simulink library "SDTlibV1"  (R2025b)
settings: Solver=VariableStepAuto  StartTime=0.0  StopTime=10.0  RelTol=1e-3
PreLoadFcn:
  | addpath(genpath('SDTfct'));
values from neighbouring files (symbols this model uses):
  pass = ra2DCMi(blk.ra)    [view_SDTlib_model.m]
undefined symbols (not defined in the file or in its folder): CMG, DAP0, DPa0, FSM, Ignew, InvDyn, InvDynAug, Jr, KIN, kinematic_model, LS, Mdyn, mnew, mp, OGnew, PMA, ra_norm, RWS, sig4, uls, ureal, uss, uw, XI
libraries: RCTblocks x470, $bdroot x4
(part 1 of 10)
settings Model: Creator=d.alazard  LastModifiedBy=ervan
settings SolverCC: AlgebraicLoopSolver=TrustRegion
settings DataIOCC: ReturnWorkspaceOutputs=off
settings DebuggingCC: UnconnectedInputMsg=warning  UnconnectedOutputMsg=warning  UnconnectedLineMsg=warning  ArithmeticOperatorsInVariantConditions=warning
settings ModelReferenceCC: EnableRefExpFcnMdlSchedulingChecks=on
settings SFSimCC: CustomCodeUndefinedFunction=UseInterfaceOnly
settings RTWCC: GPUComputeCapability=3.5  DLArmComputeVersion=19.05

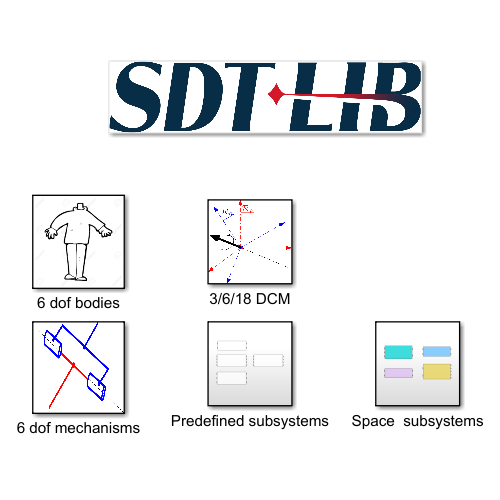
[thumbnail: Simulink's stored preview of the top-level diagram]
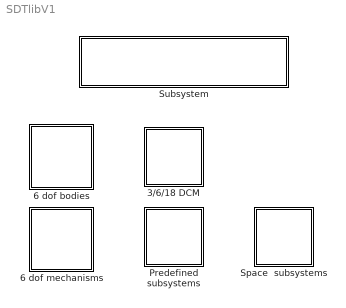
== system SDTlibV1 ==
  3/6/18 DCM : Subsystem
      mask Display: image('logoDCM.png')
  6 dof bodies : Subsystem
      mask Display: image('index.png')
  6 dof mechanisms : Subsystem
      mask Display: image('logomechanisms.png')
  Predefined subsystems : Subsystem
  Space  subsystems : Subsystem
  Subsystem : Subsystem
      mask Display: image('SDTlib_logo.png')

== system SDTlibV1/3//6//18 DCM ==
  18x18 DCM : Subsystem  mask(18x18 Direction cosine matrix (DCM)){rot=[0 1 0;-1 0 0;0 0 1], transp=off}
      mask prompts: rot "3x3 DCM"; transp "Matrix transposed"
      mask help:
      | For 6 d.o.f. body motion vector (3 translations and 3 rotations, accelerations, velocities and positions), this block Implement the 18x18 rotation matrix (or its transposed) for a given 3x3 DCM.
      |
      | Considering 2 frames R1 and  R2, the DCM between R1 and R2 is defined as the 3x3 matrix where each column is the component vector of each R2 orthogonal unit vector expressed in R1. Thus
      |
      |    [v]_R1 = DCM  * [v]_R2.
      mask init:
      | if transp,
      |     rot=rot';
      | end
      mask Help: web('Doc18dcm.html','-browser','-browser')
      mask Display:
      | disp('18x18 DCM')
      | if transp
      |     port_label('input', 1, '[.]_R1')
      |     port_label('output', 1, '[.]_R2')
      | else
      |     port_label('input', 1, '[.]_R2')
      |     port_label('output', 1, '[.]_R1')
      | end
  18x18 v-u_rotation : Subsystem  mask(18x18 rotation matrix (around a given axis)){ra=[0;-1;0], theta=ureal('alpha',0,'Range',[-pi pi]), transp=off}
      mask prompts: ra "Rotation axis (3x1 vector)"; theta "Angle (rad)"; transp "Matrix transposed"
      mask help:
      | For 6 d.o.f. body motion vector (3 translations and 3 rotations, accelerations, velocities and positions), this block Implement the 18x18 rotation matrix (or its transposed)  for a given angle around a given axis.
      |
      | Angle  (rad) can be an uncertain parameter declared with "ureal" with mode 'Range'
      | Ex: ureal('NAME',0,'Range',[-pi pi])
      | Then, ULINEARIZE will provide a model involving the block named "tan_NAME_div4".
      mask init:
      | vUrotation3x3
      mask Help: web('Doc18vurotation.html','-browser','-browser')
      mask Display:
      | disp('v-rot\n18x18')
      | if transp
      |     port_label('input', 1, '[.]_R1')
      |     port_label('output', 1, '[.]_R2')
      | else
      |     port_label('input', 1, '[.]_R2')
      |     port_label('output', 1, '[.]_R1')
      | end
  3x3 v-u_rotation : Subsystem  mask(3x3 rotation matrix (around a given axis)){ra=[0;-1;0], theta=ureal('alpha',0,'Range',[-pi pi]), transp=off}
      mask prompts: ra "Rotation axis (3x1 vector)"; theta "Angle (rad)"; transp "DCM transposed"
      mask help:
      | Implement the 3x3 direction cosine matrix (or its transposed)
      | associated to the rotation of a given angle around a given axis.
      | (DCM= matrix of coordonates of the rotated frame axes in the initial frame)
      |
      | Angle  (rad) can be an uncertain parameter declared with "ureal" with mode 'Range'
      | Ex: ureal('NAME',0,'Range',[-pi pi])
      | Then, ULINEARIZE will provide a model involving the block named "tan_NAME_div4".
      mask init:
      | vUrotation3x3
      mask Help: web('Doc3vurotation.html','-browser','-browser')
      mask Display:
      | disp('v-rot\n3x3')
      | if transp
      |     port_label('input', 1, '[.]_R1')
      |     port_label('output', 1, '[.]_R2')
      | else
      |     port_label('input', 1, '[.]_R2')
      |     port_label('output', 1, '[.]_R1')
      | end
  3x3 z-u_rotation : Subsystem  mask(3x3 rotation matrix (around 3-rd axis)){theta=ureal('alpha',0,'Range',[-180 180]), transp=off}
      mask prompts: theta "Angle (rad)"; transp "DCM transposed"
      mask help:
      | Implement the 3x3 direction cosine matrix or its transposed
      | (DCM=[cos(x)   -sin(x) 0;sin(x)  cos(x) 0;0 0 1])
      | associated to the rotation of a given angle x around the 3-rd axis.
      |
      | Angle  (rad) can be an uncertain parameter declared with "ureal" with mode 'Range'
      | Ex: ureal('NAME',0,'Range',[-pi pi])
      | Then, ULINEARIZE will provide a model involving the block named "tan_NAME_div4".
      mask init:
      | zUrotation3x3
      mask Help: web('Doc3zurotation.html','-browser','-browser')
      mask Display:
      | disp('z-rot\n3x3')
      | if transp
      |     port_label('input', 1, '[.]_R1')
      |     port_label('output', 1, '[.]_R2')
      | else
      |     port_label('input', 1, '[.]_R2')
      |     port_label('output', 1, '[.]_R1')
      | end
  6x6 DCM : Subsystem  mask(6x6 Direction cosine matrix (DCM)){rot=[0 1 0;-1 0 0;0 0 1], transp=off}
      mask prompts: rot "3x3 DCM"; transp "Matrix transposed"
      mask help:
      | For 6 d.o.f. body motion (3 translations and 3 rotations), this block Implement the 6x6 rotation matrix (or its transposed) for a given 3x3 DCM.
      |
      | Considering 2 frames R1 and  R2, the DCM between R1 and R2 is defined as the 3x3 matrix where each column is the component vector of each R2 orthogonal unit vector expressed in R1. Thus
      |
      |    [v]_R1 = DCM  * [v]_R2.
      mask init:
      | if transp,
      |     rot=rot';
      | end
      mask Help: web('Doc6dcm.html','-browser','-browser')
      mask Display:
      | disp('6x6 DCM')
      | if transp
      |     port_label('input', 1, '[.]_R1')
      |     port_label('output', 1, '[.]_R2')
      | else
      |     port_label('input', 1, '[.]_R2')
      |     port_label('output', 1, '[.]_R1')
      | end
  6x6 v-u_rotation : Subsystem  mask(6x6 rotation matrix (around a given axis)){ra=[0;-1;0], theta=ureal('alpha',0,'Range',[-pi pi]), transp=off}
      mask prompts: ra "Rotation axis (3x1 vector)"; theta "Angle (rad)"; transp "Matrix transposed"
      mask help:
      | For 6 d.o.f. body motion (3 translations and 3 rotations), this block Implement the 6x6 rotation matrix (or its transposed) for a given angle around a given axis.
      |
      | Angle  (rad) can be an uncertain parameter declared with "ureal" with mode 'Range'
      | Ex: ureal('NAME',0,'Range',[-pi pi])
      | Then, ULINEARIZE will provide a model involving the block named "tan_NAME_div4".
      mask init:
      | vUrotation3x3
      mask Help: web('Doc6vurotation.html','-browser','-browser')
      mask Display:
      | disp('v-rot\n6x6')
      | if transp
      |     port_label('input', 1, '[.]_R1')
      |     port_label('output', 1, '[.]_R2')
      | else
      |     port_label('input', 1, '[.]_R2')
      |     port_label('output', 1, '[.]_R1')
      | end
  6x6 z-u_rotation : Subsystem  mask(6x6 rotation matrix (around 3-rd axis)){theta=ureal('alpha',0,'Range',[-pi pi]), transp=off}
      mask prompts: theta "Angle (rad)"; transp "Matrix transposed"
      mask help:
      | For 6 d.o.f. body motion (3 translations and 3 rotations), this block implements the 6x6 rotation matrix (or its transposed) for a given angle around the 3-rd axis.
      |
      | Angle  (rad) can be an uncertain parameter declared with "ureal" with mode 'Range'
      | Ex: ureal('NAME',0,'Range',[-pi pi])
      | Then, ULINEARIZE will provide a model involving the block named "tan_NAME_div4".
      mask init:
      | zUrotation3x3
      mask Help: web('Doc6zurotation.html','-browser','-browser')
      mask Display:
      | disp('z-rot\n6x6')
      | if transp
      |     port_label('input', 1, '[.]_R1')
      |     port_label('output', 1, '[.]_R2')
      | else
      |     port_label('input', 1, '[.]_R2')
      |     port_label('output', 1, '[.]_R1')
      | end

== system SDTlibV1/6 dof bodies ==
  " 2 ports flexible beam" : Subsystem  mask(TITOP Model of a beam){l=ureal('lenght',1,'percent',20), s=1, rho=1, E=1, Iz=1, Iy=1, ni=0.35, xi=0.001, free=on, Won=on, uw_var=10, Nflex=4}
      mask prompts: l "lenght along x (m)"; s "cross section  (m^2)"; rho "mass density (Kg/m^3)"; E "Young modulus (N/m^2)"; Iz "second moment of area along z axis, Iz (m^4)"; Iy "second moment of area along y axis Iy, (m^4)"; ni "Poisson coefficient"; xi "damping ratio (nominal clamped-free beam)"; free "Free body at P"; uw_var "uncertainty (d_w, %)"; Nflex "number of flexible mode (Nflex, integer<=10)"
      mask help:
      | 24x24 dynamic model of a uniform beam (along x-axis) between
      |   *  wrench applied to the beam  (input) and motion vector (output) at the "child" (right) tip of the beam
      |   *  motion vector (input)  and wrench applied by the beam at the "parent" (left)  tip of the beam (output).
      | The model is expressed In the beam reference frame (0,x,y,z), see help.
      | Each parameter can be an uncertain parameter declared with "ureal".
      |
      |
      | RK: The last channel associated to parent port P can be inverted to free the body at the point P. In that case, 6 rigid modes (12 integrators) are added in the model to output the motion vector at the point P and the model becomes 36x12.
      mask init:
      | FlexibleBeam2PortAug
      mask Help: web('DocBeam.html','-browser','-browser')
      mask DialogControl Container7 Prompt: Direct uncertainties on flexible mode frequencies
      mask DialogControl Control2 Prompt: Uncertainties on physical parameters (length, mass density, ..) can create huge LFTs.
      mask DialogControl Control3 Prompt: Check this box to overwrite physical parameter uncertainties by a common relative uncertainty (d_w, %) on the first (Nflex) flexible mode frequencies of the clamped at P / free at C beam.
      mask DialogControl Control4 Prompt: The uncertain frequency is named: 'w_name_i' where:
      mask DialogControl Control5 Prompt: * 'name' is the current block name (reduced to its alphanumeric characters).
      mask DialogControl Control6 Prompt: * 'i' is the flexible mode number (increasing frequency order)
      mask Display:
      | if free
      |     disp('TITOP\n flexible beam\n (36x12)')
      | else
      |     disp('TITOP\n flexible beam\n (24x24)')
      | end
      | 
      | port_label('input', 1,'W./body,C')
      | port_label('output',1,'m_C')
      | 
      | if free
      |     port_label('input', 2,'W./body,P')
      |     port_label('output',2,'m_P')
      | else
      |     port_label('input', 2,'m_P')
      |     port_label('output',2,'Wbody/.,P')
      | end
  " N ports Nastran (free) body" : Subsystem  mask(NINOP Model of a Nastran body){fbdf='fbdf_plate', ff06='ff06_plate', P_gp=56, C_gp=[44;88;90;5], nf=10, Xi=0.001, free=on, uw_var=20, Nflex_w=3, uls_var=5, Nflex_LP=1, uev_var=0, Nflex_EV=0}
      mask prompts: fbdf "Name of the .bdf file (without extension)"; ff06 "Name of the .f06 file (without extension)"; P_gp "Node number corresponding to the point P (connection with parent body)"; C_gp "Node numbers corresponding to the points C (connections with child bodies)"; nf "Number of modes to be considered"; Xi "Common damping ratio"; free "Free body at P"; uw_var "uncertainties (%)"; Nflex_w "number of flexible modes (integer)"; uls_var "uncertainties (%)"; Nflex_LP "number of flexible modes (integer)"; uev_var "uncertainties (%)"; Nflex_EV "number of flexible modes (integer)"
      mask help:
      | NINOP (18n+6)x(6n+18) model of a flexible body at points C (connection point with the child  bodies) and point P (connection point with a parent body).
      | * 18nx6n transfer between the wrench applied to this body at the child points C  and motion vectors at these points
      | * 6x18 transfer between the motion vector at the "parent" point P  and the wrench applied by this body at this point
      | The model is expressed In the (inherit) body frame.
      |
      | Model is built from  the data provided by Patran/Nastran analysis output files.
      | Uncertainties can be added to the main parameters.
      |
      | RK: The last channel associated to parent port P can be inverted to free the body at the point P. In that case, 6 rigid modes (12 integrators) are added in the model to output the motion vector at the point P and the model becomes 18(n+1)x6(n+1).
      mask init:
      | n = length(C_gp);
      | NastranBodyNPortAugFree
      mask Help: web('DocNPortNastranBody.html','-browser','-browser')
      mask DialogControl Container2 Prompt: Main parameters
      mask DialogControl Container6 Prompt: Parametric uncertainties:
      mask DialogControl Container8 Prompt: Frequencies
      mask DialogControl Control18 Prompt: A common relative uncertainty (%) on the first flexible mode frequencies can be added (uncertainties can be changed later)
      mask DialogControl Control3 Prompt: The uncertain frequency is named: 'w_name_i' where:
      mask DialogControl Control4 Prompt: * 'name' is the current block name (reduced to its alphanumeric characters).
      mask DialogControl Control17 Prompt: * 'i' is the flexible mode number (increasing frequency order)
      mask DialogControl Container9 Prompt: Modal participation factors
      mask DialogControl Control20 Prompt: A common relative uncertainty (%) on the modal participation factors of the first flexible modes can be added (uncertainties can be changed later)
      mask DialogControl Control6 Prompt: The uncertain modal participation factor is named: 'LP_name_iXX' where:
      mask DialogControl Control7 Prompt: *  'name' is the current block name (reduced to its alphanumeric characters),
      mask DialogControl Control8 Prompt: * 'i' is the flexible mode number (increasing frequency order),
      mask DialogControl Control9 Prompt: * 'XX' = 'Tx', 'Ty', 'Tz', 'Rx', 'Ry', 'Rz'.
      mask DialogControl Container10 Prompt: Modal shapes
      mask DialogControl Control21 Prompt: A common relative uncertainty (%) on each eigen vector components at points C for the first flexible modes can be added (uncertainties can be changed later)
      mask DialogControl Control16 Prompt: WARNING: can generate very long process time !!
      mask DialogControl Control11 Prompt: The uncertain component is named: "EV_name_Cj_iXX' where:
      mask DialogControl Control12 Prompt: * 'name' is the current block name (reduced to its alphanumeric characters).
      mask DialogControl Control13 Prompt: * 'j' is the point C number,
      mask DialogControl Control14 Prompt: * 'i' is the flexible mode number (increasing frequency order),
      mask DialogControl Control15 Prompt: * 'XX' = 'Tx', 'Ty', 'Tz', 'Rx', 'Ry', 'Rz'.
      mask Display:
      | if free
      |     disp('NINOP (free)\n Nastran body\n 18(n+1)x6(n+1)')
      | else
      |     disp('NINOP (free)\n Nastran body\n (18n+6)x(6n+18)')
      | end
      | 
      | for ii=1:n
      |         port_label('input', ii,['W./body,C',num2str(ii)])
      |         port_label('output',ii,['m_C',num2str(ii)])
      | end
      | 
      | if free
      |     port_label('input', n+1,'W./body,P')
      |     port_label('output',n+1,'m_P')
      | else
      |     port_label('input', n+1,'m_P')
      |     port_label('output',n+1,'Wbody/.,P')
      | end
  " N ports flexible body" : Subsystem  mask(NINOP Model of a flexible body){M=50, J=[80 0 -0.1;0 20 22;-0.1 22 100], OG=[0;-2;0.03], OP=[0;0;0], nc=2, nf=3, zeta=0.003, OC1=[4;0;0], OC2=[0;0;0.1092], OC3=[1;1;1], OC4=[1;1;1], OC5=[1;1;1], OC6=[1;1;1], OC7=[1;1;1], OC8=[1;1;1], omega=[0.4*2*pi;0.6*2*pi;1.5*2*pi], uw_var=0, Nflex_w=0, LS=[-0.002 -1.5 -5 14 0.02 -0.01;5 1 -0.1 0 2 15;0.3 0.002 0.03 -0.02 3.2 -0.2], uls_var=0, Nflex_LP=0, EV_C=[-0.002 -1.5 -5 14 0.02 -0.01 -0.003 -1.2 -4 12 0.02 -0.02;5 1 -0.1 0 2 15 6 1/5 -0.2 1 3 16;0.3 0.002 0.03 -0.02 3.2 -0.2 0.2 0.001 0.02 -0.01 3.1 -0.1]', uev_var=0, Nflex_EV=0}
      mask prompts: M "Mass (kg)"; J "IInertia (at G, Kgm^2)"; OG "OG (3x1 vector, m)"; OP "OP (3x1 vector, m)"; nc "Number of child nodes (nc)"; nf "Number of flexible modes (nf)"; zeta "Common damping ratio"; OC1 "OC1 (3x1 vectorr: [x;y;z], m)"; OC2 "OC2 (3x1 vectorr: [x;y;z], m)"; OC3 "OC3 (3x1 vectorr: [x;y;z], m)"; OC4 "OC4 (3x1 vectorr: [x;y;z], m)"; OC5 "OC5 (3x1 vectorr: [x;y;z], m)"; OC6 "OC6 (3x1 vectorr: [x;y;z], m)"; OC7 "OC7 (3x1 vectorr: [x;y;z], m)"; OC8 "OC8 (3x1 vectorr: [x;y;z], m)"; omega "Nominal Frequencies"; uw_var "uncertainties (%)"; Nflex_w "number of flexible modes (integer)"; LS "Nominal Modal Participation Factors"; uls_var "uncertainties (%)"; Nflex_LP "number of flexible modes (integer)"; EV_C "Nominal Modal Shapes"; uev_var "uncertainties (%)"; Nflex_EV "number of flexible modes (integer)"
      mask help:
      | NINOP (18n+6)x(6n+18) model of a flexible body at points C (connection point with the child  bodies) and point P (connection point with a parent body).
      | * 18nx6n transfer between the wrenchs applied to this body at the child points C  and motion vectors at these points
      | * 6x18 transfer between the motion vector at the "parent" point P  and the wrench applied by this body at this point
      |
      | 0: the reference point
      | G: the center of mass
      | P: the connection point
      |
      | All parameters are expressed in the (inherit) body frame.
      |
      | Each parameter can be an uncertain parameter declared with "ureal"
      mask init:
      | FlexibleBodyNPortAug
      mask Help: web('Docnportflexiblebody.html','-browser','-browser')
      mask TypeOptions nc: 0 | 1 | 2 | 3 | 4 | 5 | 6 | 7 | 8
      mask DialogControl Container2 Prompt: Main parameters
      mask DialogControl Cport1 Prompt: C node #1
      mask DialogControl Cport2 Prompt: #2
      mask DialogControl Cport3 Prompt: #3
      mask DialogControl Cport4 Prompt: #4
      mask DialogControl Cport5 Prompt: #5
      mask DialogControl Cport6 Prompt: #6
      mask DialogControl Cport7 Prompt: #7
      mask DialogControl Cport8 Prompt: #8
      mask DialogControl Container6 Prompt: Flexible Modes Data:
      mask DialogControl Container8 Prompt: Frequencies
      mask DialogControl Control19 Prompt: Vector of modal frequencies: omega (nf x 1 vector, rad/s)
      mask DialogControl Control18 Prompt: A common relative uncertainty (%) on the first flexible mode frequencies can be added (uncertainties can be changed later)
      mask DialogControl Control3 Prompt: The uncertain frequency is named: 'w_name_i' where:
      mask DialogControl Control4 Prompt: * 'name' is the current block name (reduced to its alphanumeric characters).
      mask DialogControl Control17 Prompt: * 'i' is the flexible mode number (increasing frequency order)
      mask DialogControl Container9 Prompt: Modal participation factors
      mask DialogControl Control22 Prompt: Modal particiption factor: LS (nfx6 matrix, kg^0.5 for traslation dof, m.kg^0.5 for rotation dof )
      mask DialogControl Control20 Prompt: A common relative uncertainty (%) on the modal participation factors of the first flexible modes can be added (uncertainties can be changed later)
      mask DialogControl Control6 Prompt: The uncertain modal participation factor is named: 'LP_name_iXX' where:
      mask DialogControl Control7 Prompt: *  'name' is the current block name (reduced to its alphanumeric characters),
      mask DialogControl Control8 Prompt: * 'i' is the flexible mode number (increasing frequency order),
      mask DialogControl Control9 Prompt: * 'XX' = 'Tx', 'Ty', 'Tz', 'Rx', 'Ry', 'Rz'.
      mask DialogControl Container10 Prompt: Modal shapes
      mask DialogControl Control23 Prompt: Modal Shapes: EV_C (6nc x nf matrix)
      mask DialogControl Control21 Prompt: A common relative uncertainty (%) on each eigen vector components at points C for the first flexible modes can be added (uncertainties can be changed later)
      mask DialogControl Control16 Prompt: WARNING: can generate very long process time !!
      mask DialogControl Control11 Prompt: The uncertain component is named: "EV_name_Cj_iXX' where:
      mask DialogControl Control12 Prompt: * 'name' is the current block name (reduced to its alphanumeric characters).
      mask DialogControl Control13 Prompt: * 'j' is the point C number,
      mask DialogControl Control14 Prompt: * 'i' is the flexible mode number (increasing frequency order),
      mask DialogControl Control15 Prompt: * 'XX' = 'Tx', 'Ty', 'Tz', 'Rx', 'Ry', 'Rz'.
      mask Display:
      | disp('N-port\n flexible body\n (18n+6)x(6n+18)')
      | 
      | if n~=0
      | for ii=1:n
      |         port_label('input', ii,['W./body,C',num2str(ii)])
      |         port_label('output',ii,['m_C',num2str(ii)])
      | end
      | end
      | 
      | port_label('input', n+1,'m_P')
      | port_label('output',n+1,'Wbody/.,P')
  1 port Nastran body : Subsystem  mask(One port Nastran body){ff06='ff06_plate', nf=4, xi=0.001, dw=[20;10;0;0]}
      mask prompts: ff06 "Name of the .f06 file (without extension)"; nf "Number of modes to be considered (nf)"; xi "Common damping ratio"; dw "uncertainties (%):"
      mask help:
      | Dynamic model of a flexible body at point P (connection point with a parent body):
      | 6x18 transfer between accelaretion twist at P and wrench applied by this body at P.
      | The model is expressed in the (inherit) body frame.
      |
      | Model is built from  the data provided by Patran/Nastran analysis output files.
      mask init:
      | NastranBody1Port
      mask Help: web('Doc1PortNastranBody.html','-browser','-browser')
      mask DialogControl ParameterGroupVar Prompt: Main Parameters
      mask DialogControl Container6 Prompt: Uncertainties on flexible mode frequencies (%):
      mask DialogControl Control5 Prompt: * a common value or a vector with nf components (increasing frequency order)
      mask DialogControl Control6 Prompt: * for the flexible mode i (1,...,nf), the uncertain frequency is named:
      mask DialogControl Control7 Prompt: 'w_name_i' where 'name' is the current block name (reduced to its alphanumeric characters).
      mask Display:
      | disp('One-port\n Nastran body\n (6x18)')
      | port_label('input', 1, 'm')
      | port_label('output', 1, 'Wbody/.')
  1 port flexible body : Subsystem  AncestorBlock=SDTlibV2/6 dof bodies/1 port flexible body  mask(One-port flexibe body (6x18)){m=1, Ig=zeros(3), OG=[0;0;0], OP=[0;0;0], xi=0.001, uw=zeros(10,1), uls=zeros(10,6)}
      mask prompts: m "Mass (Kg)"; Ig "Inertia (at G, Kgm^2)"; OG "OG (3x1 vector, m)"; OP "OP (3x1 vector, m)"; xi "Common damping ratio"; uw "Frequencies (rad/s)"; uls "Modal participation factors matrix"
      mask help:
      | 6x18 dynamic model between the motion vector and the wrench applied by this body at point P (connection point with a parent body).
      | Dynamic model of a flexible body at point P (connection point with  parent body).
      |
      | 0: the reference point
      | G: the center of mass
      | P: the connection point
      |
      | All parameters are expressed in the (inherit) body frame.
      |
      | Each parameter can be an uncertain parameter declared with "ureal"
      mask init:
      | FlexBody1Port
      mask Help: web('Doconeportflexiblebody.html','-browser','-browser')
      mask DialogControl ParameterGroupVar Prompt: Main parameters
      mask Display:
      | disp('One-port\n flexible body\n (6x18)')
      | port_label('input', 1, 'm')
      | port_label('output', 1, 'Wbody/.')
  Multi in/out-port flexible body : Subsystem  mask(Multi-port flexible body){M=[eye(6) 0.1*[1 0 0 0;0 1 0 0;0 0 1 0;0 0 0 1;1 0 1 0;0 1 0 1];0.1*[1 0 0 0;0 1 0 0;0 0 1 0;0 0 0 1;1 0 1 0;0 1 0 1]' eye(4)], K=[zeros(6,10);zeros(4,6) diag([1 2 3 4])], D=[zeros(6,10); zeros(4,6) 0.005*eye(4)], PHIin=[eye(6) eye(6) kinematic_model([0;0;0],[0;1;1]);zeros(4,6) [eye(4) zeros(4,2)] [zeros(4,1) eye(4) zeros(4,1)]], PHIout=[eye(6) eye(6) eye(6) eye(6);zeros(4,6) [eye(4) zeros(4,2)] [zeros(4,1) eye(4) zeros(4,1)] [zeros(4,2) eye(4)]]', free=on, reduction=on, n=2}
      mask prompts: M "Mass Matrix (M)"; K "Stiffness Matrix (K)"; D "Damping Matrix (D)"; PHIin "Input Projection Matrix (PHIin)"; PHIout "Output Projection Matrix (PHIout)"; free "Free body at P"; reduction "Model reduction"; n "number of flexible modes"
      mask help:
      | (18no-12)x(6ni+12) dynamic model of a flexiible body defined by M, K, D, PHIin and PHIout matrices
      |
      | P: the parent point (the cantilevered point of the body).
      | Bi (i=1,..., ni): the child points where are applied external wrenches,
      | Ci (i=1,...,no): the child points where are measured accelerations
      |
      | RK: The last channel associated to parent port P can be inverted to free the body at the point P. In that case, 6 rigid modes (12 integrators) are added in the model to output the motion vector at the point P  18(no+1)x6(ni+1)
      |
      | The model can also be reduced.
      mask init:
      | Multi_IO_FlexibleBodyRedAug
      mask Help: web('DocIOportFlexibleBodyRed.html','-browser','-browser')
      mask DialogControl ParameterGroupVar Prompt: Main parameters
      mask DialogControl Container4 Prompt: Model order = 2 * number of flexible modes
      mask Display:
      | disp('Multi in/out-port\n flexible body\n (M,K,D,\n PHIin,PHIout)')
      | for ii=1:nB
      |     port_label('input', ii,['W./body,B',num2str(ii)])
      | end
      | for ii=1:nC
      |     port_label('output',ii,['m_C',num2str(ii)])
      | end
      | if free,
      |     port_label('input', nB+1,'W./body,P')
      |     port_label('output',nC+1,'m_P')
      | else
      |     port_label('output',nC+1,'Wbody/.,P')
      |     port_label('input', nB+1,'m_P')
      | end
  Multi port flexible body : Subsystem  mask(Multi-port flexible body){M=[eye(6) 0.1*[1 0 0 0;0 1 0 0;0 0 1 0;0 0 0 1;1 0 1 0;0 1 0 1];0.1*[1 0 0 0;0 1 0 0;0 0 1 0;0 0 0 1;1 0 1 0;0 1 0 1]' eye(4)], K=[zeros(6,10);zeros(4,6) diag([1 2 3 4])], D=[zeros(6,10); zeros(4,6) 0.005*eye(4)], PHI=[eye(6) eye(6) eye(6) kinematic_model([0;0;0],[1;0;1]);zeros(4,6) [eye(4) zeros(4,2)] [zeros(4,2) eye(4)] [zeros(4,1) eye(4) zeros(4,1)]], free=off, reduction=on, n=2}
      mask prompts: M "Mass Matrix (M)"; K "Stiffness Matrix (K)"; D "Damping Matrix (D)"; PHI "Projection Matrix (PHI)"; free "Free body at P"; reduction "Model reduction:"; n "number of flexible modes"
      mask help:
      | (18n-12)x(6n+12) dynamic TITOP model of a flexiible body defined by M, K, D and PHI matrices
      |
      | P: the parent point (the cantilevered point of the body).
      | Ci: the child points
      |
      | RK: The last channel associated to parent port P can be inverted to free the body at the point P. In that case, 6 rigid modes (12 integrators) are added in the model to output the motion vector at the point P and the model becomes 18nx6n.
      |
      | The model can also be reduced.
      mask init:
      | MultiPortFlexibleBodyRedAug
      mask Help: web('DocNPortFlexibleBodyRed.html','-browser','-browser')
      mask DialogControl ParameterGroupVar Prompt: Main parameters
      mask DialogControl Container1 Prompt: Model order = 2 * number of flexible modes
      mask Display:
      | disp('Multi-port\n flexible body\n (M,K,D,PHI)')
      | for ii=1:nC
      |     port_label('input', ii,['W./body,C',num2str(ii)])
      |     port_label('output',ii,['m_C',num2str(ii)])
      | end
      | if free,
      |     port_label('input', nC+1,'W./body,P')
      |     port_label('output',nC+1,'m_P')
      | else
      |     port_label('output',nC+1,'Wbody/.,P')
      |     port_label('input', nC+1,'m_P')
      | end
  Multi port rigid body : Subsystem  mask(Multi-port rigid body (18(n-1)+6]x[6(n-1)+18])){m=ureal('Mass',1000,'percent',10);, Ig=[400 -10 3;-10 ureal('Iyy',1000,'percent',10) -40;3 -40 1000], OG=[1;0;0], n=3, numinv=3, OP1=[0;0;0], OP2=[2;0;0], OP3=[ureal('P3_y',1,'percent',10);0;0], OP4=[0;0;0], OP5=[0;0;0]}
      mask prompts: m "Mass (Kg)"; Ig "Inertia (at G, Kg m^2)"; OG "OG (3x1 vector, m)"; n "Number of ports"; numinv "The single parent port"; OP1 "OP1 (3x1 vector, m)"; OP2 "OP2 (3x1 vector, m)"; OP3 "OP3 (3x1 vector, m)"; OP4 "OP4 (3x1 vector, m)"; OP5 "OP5 (3x1 vector,m)"
      mask help:
      | [18(n-1)+6]x[6(n-1)+18] dynamic model of a rigid body at n given points (ports) between:
      | * the wrenches applied at the n-1 child ports and  the motion vector at a single parent port (inputs).
      | * the motions vectors at the  n-1 child ports and the wrench applied by the rigid body at the parent port (output)
      |
      | 0: the reference point
      | G: the center of mass
      | Pi (i=1:n): the n given connection points (n<6).
      |
      | All parameters are expressed in the body frame.
      | Each parameter can be an uncertain parameter declared with "ureal"
      |
      | The 6x18 channel associated to the single parent port can be any of the ports.
      mask init:
      | MultiPortRigidBodyAug
      mask Help: web('Docmultiportrigidbody.html','-browser','-browser')
      mask TypeOptions n: 1 | 2 | 3 | 4 | 5
      mask TypeOptions numinv: 1 | 2 | 3 | 4 | 5
      mask DialogControl ParameterGroupVar Prompt: Main parameters
      mask DialogControl port1 Prompt: Port #1
      mask DialogControl port2 Prompt: #2
      mask DialogControl port3 Prompt: #3
      mask DialogControl port4 Prompt: #4
      mask DialogControl port5 Prompt: #5
      mask Display:
      | disp('Multi-port\n rigid body\n [18(n-1)+6]x[6(n-1)+18]')
      | if n==1,
      |     if numinv==1,
      |         port_label('input', 1,'m_P')
      |         port_label('output',1,'Wbody/.,P')
      |     else
      |         port_label('input', 1,'W./body,P')
      |         port_label('output',1,'m_P')
      |     end
      | else
      |     for ii=1:n
      |         if numinv==ii,
      |             port_label('output',ii,['Wbody/.,P',num2str(ii)])
      |             port_label('input', ii,['m_P',num2str(ii)])
      |         else
      |             port_label('input', ii,['W./body,P',num2str(ii)])
      |             port_label('output',ii,['m_P',num2str(ii)])
      |         end
      |     end
      | end
  Multi port rigid free body : Subsystem  mask(Multi-port rigid body (18nx6n)){m=ureal('Mass',1000,'percent',10);, Ig=[400 -10 3;-10 ureal('Iyy',1000,'percent',10) -40;3 -40 1000], OG=[1;0;0], n=3, OP1=[0;0;0], OP2=[2;0;0], OP3=[ureal('P3_y',1,'percent',10);0;0], OP4=[0;0;0], OP5=[0;0;0]}
      mask prompts: m "Mass (Kg)"; Ig "Inertia (at G, Kg m^2)"; OG "OG (3x1 vector, m)"; n "Number of ports"; OP1 "OP1 (3x1 vector, m)"; OP2 "OP2 (3x1 vector, m)"; OP3 "OP3 (3x1 vector, m)"; OP4 "OP4 (3x1 vector, m)"; OP5 "OP5 (3x1 vector,m)"
      mask help:
      | 18nx6n dynamic model of a rigid body at n given points (ports) between wrenches applied at the n points (input) and the motions vectors at these points (output).
      |
      | 0: the reference point
      | G: the center of mass
      | Pi (i=1:n): the n given connection points (n<6).
      |
      | All parameters are expressed in the body frame.
      | Each parameter can be an uncertain parameter declared with "ureal"
      mask init:
      | MultiPortRigidFreeBody
      mask Help: web('Docmultiportrigidbase.html','-browser','-browser')
      mask TypeOptions n: 1 | 2 | 3 | 4 | 5
      mask DialogControl ParameterGroupVar Prompt: Main parameters
      mask DialogControl port1 Prompt: Port #1
      mask DialogControl port2 Prompt: #2
      mask DialogControl port3 Prompt: #3
      mask DialogControl port4 Prompt: #4
      mask DialogControl port5 Prompt: #5
      mask Display:
      | disp('Multi-port\n rigid free body\n (18nx6n)')
      | for ii=1:n
      |     port_label('input', ii,['W_{./body,P',num2str(ii),'}'],'interpreter','tex')
      |     port_label('output',ii,['m_{P',num2str(ii),'}'],'interpreter','tex')
      | end
  massless connection body : Subsystem  mask(Massless multi_port [6+18(n-1)]x[6(n-1)+18]){n=4, numinv=3, OP1=[0;0;0], OP2=[2;0;0], OP3=[ureal('P3_y',1,'percent',10);0;0], OP4=[0;0;0], OP5=[0;0;0], OP6=[0;0;0], OP7=[0;0;0]}
      mask prompts: n "Number of ports"; numinv "Port (point) Pj: j="; OP1 "OP1 (3x1 vector, m)"; OP2 "OP2 (3x1 vector, m)"; OP3 "OP3 (3x1 vector, m)"; OP4 "OP4 (3x1 vector, m)"; OP5 "OP5 (3x1 vector,m)"; OP6 "OP6 (3x1 vector,m)"; OP7 "OP7 (3x1 vector,m)"
      mask help:
      | Massless body to transport wrenches and acceleration twists:
      | [6+18(n-1)]x[6(n-1)+18] gain from:
      |  * the motion vector at one point Pj; i.e. the parent port,
      |  * the wrenches applied to this massless body at the n-1 points Pi (i=1,..n, except j); i.e. the child ports
      | to:
      |  * the wrench applied at point Pj by this massless body,
      |  * the motion vectors at the other n-1  points Pi (i=1,..n, except j).
      |
      | 0: the reference point
      | Pi (i=1:n): the n given connection points or ports (1<n<8).
      |
      | All parameters are expressed in the body frame.
      | Each parameter can be an uncertain parameter declared with "ureal"
      mask init:
      | MasslessConnectionBodyAug
      mask Help: web('DocMassLessBody.html','-browser','-browser')
      mask TypeOptions n: 2 | 3 | 4 | 5 | 6 | 7
      mask TypeOptions numinv: 1 | 2 | 3 | 4 | 5 | 6 | 7
      mask DialogControl ParameterGroupVar Prompt: Main parameters
      mask DialogControl port1 Prompt: Port #1
      mask DialogControl port2 Prompt: #2
      mask DialogControl port3 Prompt: #3
      mask DialogControl port4 Prompt: #4
      mask DialogControl port5 Prompt: #5
      mask DialogControl port6 Prompt: #6
      mask DialogControl port7 Prompt: #7
      mask Display:
      | disp('Massless\n connection body\n [6+18(n-1)]x[6(n-1)+18]')
      | for ii=1:n+1
      |     if numinv==ii,
      |         port_label('output',ii,['Wbody/.,P',num2str(ii)])
      |         port_label('input', ii,['m_P',num2str(ii)])
      |     else
      |         port_label('input', ii,['W./body,P',num2str(ii)])
      |         port_label('output',ii,['m_P',num2str(ii)])
      |     end
      | end
  multi-port FEM Kirchhoff plate : Subsystem  mask(Multi-port flexible plate (18nC+6nP)x(6nC+18nP)){lx=1, ly=1, t=0.01, rho=2700, E=70e9, ni=0.35, xi=0.001, nx=4, ny=4, i_nP=2, i_nC=3, P1=1, P2=20, P3=25, P4=20, C1=5, C2=25, C3=8, C4=1, C5=1, C6=1, C7=1, C8=1, RedSlowOn=off, RedFastOn=on, w_trunc=5000, uw_var=10, Nflex=3}
      mask prompts: lx "lenght along x (m)"; ly "length along y (m)"; t "thickness (m)"; rho "mass density (Kg/m^3)"; E "Young modulus (N/m^2)"; ni "Poisson coefficient"; xi "damping coefficient"; nx "number of elements along x (integer)"; ny "number of elements along y (integer)"; i_nP "number (nP) of parent (P) nodes (<5)"; i_nC "number (nC) of child (C) nodes"; P1 "P1 (integer)"; P2 "P2 (integer)"; P3 "P3 (integer)"; P4 "P4 (integer)"; C1 "C1 (integer)"; C2 "C2 (integer)"; C3 "C3 (integer)"; C4 "C4 (integer)"; C5 "C5 (integer)"; C6 "C6 (integer)"; C7 "C7 (integer)"; C8 "C8 (inreger)"; RedSlowOn "Reduction of the 6*(nP-1) poles at 0 (due to loop closure constraints when nP>1)."; RedFastOn "Reduction of fast flexible modes:"; w_trunc "with a frequency (rad/s) >"; uw_var "uncertainty (%)"; Nflex "number of flexible modes (Nf, integer)"
      mask help:
      | (18nC+6nP)x(6nC+18nP) multi-port model of a uniform plate (in the x-y plane) between
      |   *  wrenches applied to the plate at the given nC child nodes (input) and motion vectors at these child nodes (output)
      |   *  motion vectors at the nP parent nodes (input)  and wrenches applied by this plate at these parent nodes (output)
      |  dynamic model of a uniform flexible plate (in the x-y plane),
      | in the plate reference frame (0,x,y,z)
      |
      | The plate is defined by:
      | * 0<x<lx
      | * 0<y<ly
      | * -t/2<z<t/2
      |
      | This model is based on a finite element apprach using (nx x ny) elements (nx and ny elements along x and y axes, respectiveley).  The parents and child nodes must be specified by their indexes in the list of the (nx+1)x(n
      | y+1) nodes defined by:
      |  * node 1 is the point (0,0) of the plate,
      |  * node nx+1 is the point (lx,0) of the plate,
      |  * node nx+2 is the point (0, ly/ny) of the plate,
      |  * node 2*(nx+1) is the point (lx,ly/ny) of the plate,
      |  * ....
      |  * node j*(nx+1) is the point (lx,(j-1)*ly/ny) of the plate,
      |  * node j*(nx+1)+1 is the point (0, j*ly/ny) of the plate,
      |  * ...
      |  * node (ny+1)*(nx+1) is the point (lx,ly) of the plate.
      |
      | This block can also performed optional model reductions:
      |    * reduction of the 6*(nP-1) poles at 0 due to loop closure constraints,
      |    * reduction of the flexible modes which a frequnecy (rad/s) greated than a specified value.
      |
      | See the inline help for more details.
      |
      | All parameters are expressed in the plate reference fram.
      | Dynamics in translations along x and y and rotation around z are assumed rigid.
      mask init:
      | MultiPortFEMKirchhoffPlateAug
      mask Help: web('DocPlate_Kirchhoff.html','-browser','-browser')
      mask TypeOptions i_nP: 0 | 1 | 2 | 3 | 4
      mask TypeOptions i_nC: 0 | 1 | 2 | 3 | 4 | 5 | 6 | 7 | 8
      mask DialogControl ParameterGroupVar Prompt: Main parameters
      mask DialogControl Pport1 Prompt: P node #1
      mask DialogControl Pport2 Prompt: #2
      mask DialogControl Pport3 Prompt: #3
      mask DialogControl Pport4 Prompt: #4
      mask DialogControl Cport1 Prompt: C node #1
      mask DialogControl Cport2 Prompt: #2
      mask DialogControl Cport3 Prompt: #3
      mask DialogControl Cport4 Prompt: #4
      mask DialogControl Cport5 Prompt: #5
      mask DialogControl Cport6 Prompt: #6
      mask DialogControl Cport7 Prompt: #7
      mask DialogControl Cport8 Prompt: #8
      mask DialogControl Reduction Prompt: Optional Reduction
      mask DialogControl Container21 Prompt: Parametric uncertainties
      mask DialogControl Control2 Prompt: The uncertain parameters are the first Nf cantilevered frequencies of the plate when it is clamped at the first parent node (P1) or the last child node CnC when the number of parent nodes is null.
      mask DialogControl Control3 Prompt: The uncertain frequency is named: 'w_name_i' where:
      mask DialogControl Control4 Prompt: * 'name' is the current block name (reduced to its alphanumeric characters).
      mask DialogControl Control5 Prompt: * 'i' is the flexible mode number (increasing frequency order)
      mask Display:
      | disp('NINOP FEM\n Kirchhoff plate\n (18nC+6nP)x(6nC+18nP)')
      | if nC~=0
      |     for ii=1:nC
      |         port_label('input', ii, ['W./body,C',num2str(ii)])
      |         port_label('output',ii,['m_C',num2str(ii)])
      |     end
      | end
      | if nP~=0
      |     for ii=1:nP
      |         port_label('input', nC+ii, ['m_P',num2str(ii)])
      |         port_label('output',nC+ii,['Wbody/.,P',num2str(ii)])
      |     end
      | end
  multi-port flexible plate : Subsystem  mask(Multi-port flexible plate (18nC+6nP)x(6nC+18nP)){lx=4.14, ly=2.2, t=0.01, rho=474, E=44e9, ni=0.35, xi=0, i_nP=1, i_nC=3, OP1=[0;1.1;0], OP2=[4.14;1.1;0], OP3=[4.14;0;0], OP4=[4.14;2.2;0], OC1=[4.14;2.2;0], OC2=[0;0;0], OC3=[4.14;0;0], OC4=[4.14;2.2;0], OC5=[4.14;1.1;0], OC6=[0;1.1;0], OC7=[0;0;0], OC8=[0;0;0], RedSlowOn=off, uw_var=5, Nflex=3}
      mask prompts: lx "lenght along x (m)"; ly "length along y (m)"; t "thickness (m)"; rho "Mass density (Kg/m^3)"; E "Young modulus (N/m^2)"; ni "Poisson coefficient"; xi "damping coefficient"; i_nP "Number of parent (P) nodes (<5)"; i_nC "Number of child (C) nodes"; OP1 "OP1 (3x1 vector: [x;y;0], m)"; OP2 "OP2 (3x1 vectorr: [x;y;0], m)"; OP3 "OP3 (3x1 vectorr: [x;y;0], m)"; OP4 "OP4 (3x1 vectorr: [x;y;0], m)"; OC1 "OC1 (3x1 vectorr: [x;y;0], m)"; OC2 "OC2 (3x1 vectorr: [x;y;0], m)"; OC3 "OC3 (3x1 vectorr: [x;y;0], m)"; OC4 "OC4 (3x1 vectorr: [x;y;0], m)"; OC5 "OC5 (3x1 vectorr: [x;y;0], m)"; OC6 "OC6 (3x1 vectorr: [x;y;0], m)"; OC7 "OC7 (3x1 vector: [x;y;0],m)"; OC8 "OC8 (3x1 vector [x;y;0], m)"; RedSlowOn "Reduction of the 6*(nP-1) poles at 0 (due to loop closure constraints when nP>1)."; uw_var "uncertainty (%)"; Nflex "number of flexible modes (Nf, integer)"
      mask help:
      | (18nC+6nP)x(6nC+18nP) multi-port model of a uniform plate (in the x-y plane) between
      |   *  wrenches applied to the plate at the given nC child nodes (input) and motion vectors at these child nodes (output)
      |   *  motion vectors at the nP parent nodes (input)  and wrenches applied by this plate at these parent nodes (output)
      |  dynamic model of a uniform flexible plate (in the x-y plane),
      | in the plate reference frame (0,x,y,z)
      |
      | The plate is defined by:
      | * 0<x<lx
      | * 0<y<ly
      | * -t/2<z<t/2
      |
      | All parameters are expressed in the plate reference frame.
      | Dynamics in translations along x and y and rotation around z are assumed rigid.
      mask init:
      | MultiPortFlexiblePlateAug
      mask Help: web('DocPlate_joly.html','-browser','-browser')
      mask TypeOptions i_nP: 0 | 1 | 2 | 3 | 4
      mask TypeOptions i_nC: 0 | 1 | 2 | 3 | 4 | 5 | 6 | 7 | 8
      mask DialogControl ParameterGroupVar Prompt: Main parameters
      mask DialogControl Pport1 Prompt: P node #1
      mask DialogControl Pport2 Prompt: #2
      mask DialogControl Pport3 Prompt: #3
      mask DialogControl Pport4 Prompt: #4
      mask DialogControl Cport1 Prompt: C node #1
      mask DialogControl Cport2 Prompt: #2
      mask DialogControl Cport3 Prompt: #3
      mask DialogControl Cport4 Prompt: #4
      mask DialogControl Cport5 Prompt: #5
      mask DialogControl Cport6 Prompt: #6
      mask DialogControl Cport7 Prompt: #7
      mask DialogControl Cport8 Prompt: #8
      mask DialogControl Reduction Prompt: Optional Reduction
      mask DialogControl Container19 Prompt: Parametric uncertainties
      mask DialogControl Control8 Prompt: The uncertain parameters are the first Nf cantilevered frequencies of the plate when it is clamped at the first parent node (P1) or the last child node when the number of parent nodes is null.
      mask DialogControl Control4 Prompt: The uncertain frequency is named: 'w_name_i' where:
      mask DialogControl Control5 Prompt: * 'name' is the current block name (reduced to its alphanumeric characters).
      mask DialogControl Control6 Prompt: * 'i' is the flexible mode number (increasing frequency order)
      mask Display:
      | disp('NINOP\n flexible plate\n (18nC+6nP)x(6nC+18nP)')
      | if nC~=0
      |     for ii=1:nC
      |         port_label('input', ii, ['W./body,C',num2str(ii)])
      |         port_label('output',ii,['m_C',num2str(ii)])
      |     end
      | end
      | if nP~=0
      |     for ii=1:nP
      |         port_label('input', nC+ii, ['m_P',num2str(ii)])
      |         port_label('output',nC+ii,['Wbody/.,P',num2str(ii)])
      |     end
      | end
